simulink model "KP_sim_test"  (R2024b)
settings: Solver=VariableStepAuto  StartTime=0.0  StopTime=150  MaxStep=1e-3  RelTol=1e-3
undefined symbols (not defined in the file or in its folder): DiscIntNeverNeededParam
libraries: simulink_extras x3
settings Model: Creator=Pedro  LastModifiedBy=Pedro

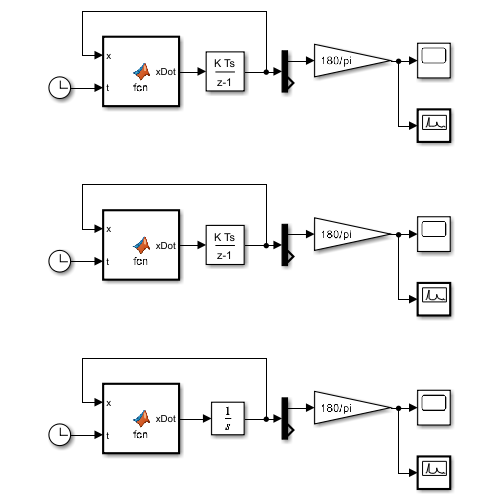
[thumbnail: Simulink's stored preview of the top-level diagram]
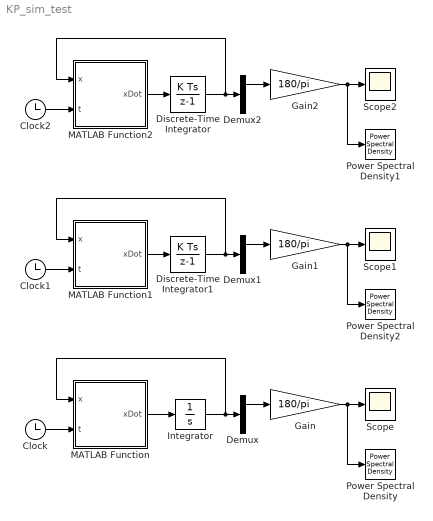
== system KP_sim_test ==
  Clock : Clock
  Clock1 : Clock
  Clock2 : Clock
  Demux : Demux  Outputs=2
  Demux1 : Demux  Outputs=2
  Demux2 : Demux  Outputs=2
  Discrete-Time Integrator : DiscreteIntegrator  InitialCondition=pi/180*[10;0]  SampleTime=0.00001  ICPrevOutput=DiscIntNeverNeededParam  ICPrevScaledInput=DiscIntNeverNeededParam
  Discrete-Time Integrator1 : DiscreteIntegrator  InitialCondition=pi/180*[10;0]  SampleTime=0.03  ICPrevOutput=DiscIntNeverNeededParam  ICPrevScaledInput=DiscIntNeverNeededParam
  Gain : Gain  Gain=180/pi
  Gain1 : Gain  Gain=180/pi
  Gain2 : Gain  Gain=180/pi
  Integrator : Integrator  InitialCondition=pi/180*[10;0]
  MATLAB Function : MATLAB Function  TreatAsAtomicUnit=on
  MATLAB Function1 : MATLAB Function  TreatAsAtomicUnit=on
  MATLAB Function2 : MATLAB Function  TreatAsAtomicUnit=on
  Power Spectral Density : simulink_extras/Additional Sinks/Power Spectral Density  npts=512  fftpts=512  HowOften=16  sampleT=0.02
  Power Spectral Density1 : simulink_extras/Additional Sinks/Power Spectral Density  npts=512  fftpts=512  HowOften=16  sampleT=0.02
  Power Spectral Density2 : simulink_extras/Additional Sinks/Power Spectral Density  npts=512  fftpts=512  HowOften=16  sampleT=0.02
  Scope : Scope
  Scope1 : Scope
  Scope2 : Scope
  wires:
  MATLAB Function/1(xDot) -> Integrator/1
  Integrator/1 -> MATLAB Function/1(x), Demux/1
  Clock/1 -> MATLAB Function/2(t)
  Gain/1 -> Power Spectral Density/1, Scope/1
  Demux/1 -> Gain/1
  Demux1/1 -> Gain1/1
  Discrete-Time Integrator1/1 -> MATLAB Function1/1(x), Demux1/1
  Clock1/1 -> MATLAB Function1/2(t)
  Gain1/1 -> Power Spectral Density2/1, Scope1/1
  MATLAB Function1/1(xDot) -> Discrete-Time Integrator1/1
  Demux2/1 -> Gain2/1
  Discrete-Time Integrator/1 -> MATLAB Function2/1(x), Demux2/1
  Clock2/1 -> MATLAB Function2/2(t)
  Gain2/1 -> Power Spectral Density1/1, Scope2/1
  MATLAB Function2/1(xDot) -> Discrete-Time Integrator/1

== matlab function KP_sim_test/MATLAB Function1 ==
  settings: updateMethod=CONTINUOUS  sampleTime=1e-3
  data: x input; xDot output; t input
function xDot = fcn(x,t)

% Physical parameters
g = 9.81;       % gravitational acceleration [m/s^2]
L = 1;        % pendulum length [m]
zeta = 0.01;    % damping ratio [-]
A = 0.36;
frequencyHz = 5.5;

% Natural and excitation frequencies
Omega = sqrt(g/L);
omega = 2*pi*frequencyHz;

% Base acceleration amplitude
% A is the base displacement amplitude [m]
a0 = A*omega^2;

% Periodic excitation
phi = cos(omega*t);

% States
theta = x(1);
thetaDot = x(2);

% Nonlinear inverted-pendulum equation
thetaDDot = -2*zeta*Omega*thetaDot ...
    - (-Omega^2 + (a0/L)*phi)*sin(theta);

% State derivative
xDot = [thetaDot; thetaDDot];

end

== matlab function KP_sim_test/MATLAB Function ==
  settings: updateMethod=CONTINUOUS  sampleTime=1e-3
  data: x input; xDot output; t input
function xDot = fcn(x,t)

% Physical parameters
g = 9.81;       % gravitational acceleration [m/s^2]
L = 1;        % pendulum length [m]
zeta = 0.01;    % damping ratio [-]
A = 0.36;
frequencyHz = 5.5;

% Natural and excitation frequencies
Omega = sqrt(g/L);
omega = 2*pi*frequencyHz;

% Base acceleration amplitude
% A is the base displacement amplitude [m]
a0 = A*omega^2;

% Periodic excitation
phi = cos(omega*t);

% States
theta = x(1);
thetaDot = x(2);

% Nonlinear inverted-pendulum equation
thetaDDot = -2*zeta*Omega*thetaDot ...
    - (-Omega^2 + (a0/L)*phi)*sin(theta);

% State derivative
xDot = [thetaDot; thetaDDot];

end

== matlab function KP_sim_test/MATLAB Function2 ==
  settings: updateMethod=CONTINUOUS  sampleTime=1e-3
  data: x input; xDot output; t input
function xDot = fcn(x,t)

% Physical parameters
g = 9.81;       % gravitational acceleration [m/s^2]
L = 1;        % pendulum length [m]
zeta = 0.01;    % damping ratio [-]
A = 0.36;
frequencyHz = 5.5;

% Natural and excitation frequencies
Omega = sqrt(g/L);
omega = 2*pi*frequencyHz;

% Base acceleration amplitude
% A is the base displacement amplitude [m]
a0 = A*omega^2;

% Periodic excitation
phi = cos(omega*t);

% States
theta = x(1);
thetaDot = x(2);

% Nonlinear inverted-pendulum equation
thetaDDot = -2*zeta*Omega*thetaDot ...
    - (-Omega^2 + (a0/L)*phi)*sin(theta);

% State derivative
xDot = [thetaDot; thetaDDot];

end
